simulink model "GolfSwing3D_KineticallyDrivenBlockCountStrip"  (R2024b)
settings: Solver=VariableStepAuto  StartTime=0.0  StopTime=StopTime  MaxStep=0.001  RelTol=1e-3
model workspace: external: MAT-File 3DModelInputs.mat (data not in the file)
undefined symbols (not defined in the file or in its folder): GripStrength, KillswitchFinalValue, KillswitchInitialValue, KillswitchStepTime, LeftLowerArmLength, PlaneTilt, RightLowerArmLength, UpperTorsoLength, X, Y, Z
libraries: nesl_utility x361, sm_lib x136, matrix_library x11, fl_lib x2, simulink x1
(part 12 of 13)

== matlab function GolfSwing3D_KineticallyDrivenBlockCountStrip/RE Input Function/Right Elbow Input Torque ==
  data: Time input; Killswitch input; JointTorqueRE output; REPositionInput output; REInputB parameter; REPositionSetpoint parameter; GlobalGain parameter; REDampening parameter; ModelingMode parameter; GlobalPCGain parameter; GlobalVCGain parameter; DampeningGlobalGain parameter; TargetImpactTime parameter; KinematicMode parameter; REAo parameter; REStartPosition parameter; REStartVelocity parameter; REVCGain parameter; TargetREVelocity parameter; TargetREPosition parameter; REPositionGain parameter; REInputC parameter; RETimeGain parameter; REVelocityInput output; REAccelerationInput output; REConstant parameter; REPosition input; REVelocity input; ZVCFRETorque parameter; REPCGain parameter; REInputA parameter; REAf parameter; REInputD parameter; REInputE parameter; REInputF parameter; REInputG parameter
function [JointTorqueRE,REPositionInput,REVelocityInput,...
    REAccelerationInput]  = fcn(Time,Killswitch,...
    REInputB,REPositionSetpoint,GlobalGain,...
    REDampening, ModelingMode,GlobalPCGain, GlobalVCGain,...
    DampeningGlobalGain,TargetImpactTime,KinematicMode, REAo,REStartPosition,...
    REStartVelocity,REVCGain,...
    TargetREVelocity,TargetREPosition, ...
    REPositionGain,REInputC,...
    RETimeGain, REConstant, REPosition,REVelocity, ZVCFRETorque, REPCGain,...
    REInputA,REAf,REInputD, REInputE, REInputF, REInputG)

%Tau=Time/TargetImpactTime;
t=Time;

% %%%%%%%%%%%%%%%%%%%%%%%%%%%%%%%%%%%%%%%%%%%
% % Kinetic Input Selection and Calculation
% %%%%%%%%%%%%%%%%%%%%%%%%%%%%%%%%%%%%%%%%%%%

if ModelingMode==0
    % Values are all set to zero.
    JointTorqueRE=0;
elseif ModelingMode==1
    % Control based strategy. Values are based on difference in value
    % between the current state and desired state.
    % RE Joint Rotational Deltas
    DeltaREPosition=REPosition-TargetREPosition;
    DeltaREVelocity=REVelocity-TargetREVelocity;
    % Control Based Strategy
    JointTorqueRE=DeltaREPosition*REPCGain*GlobalPCGain-DeltaREVelocity*REVCGain*GlobalVCGain-DampeningGlobalGain*REDampening*REVelocity;
elseif ModelingMode==2
    % Forward Dynamics Based Strategy. Values are computed based on a
    % polynomial and a combination of dampening and position gained
    % factors.
    JointTorqueRE=Killswitch*GlobalGain*(REConstant+RETimeGain*Time-REPositionGain*(REPosition-REPositionSetpoint)...
    -REDampening*REVelocity);
elseif ModelingMode==3
    JointTorqueRE=HexPolyInputFunction(REInputA,REInputB,REInputC,REInputD,REInputE,REInputF,REInputG,Time)*Killswitch;
else
    %ZVCF Based Joint Torques. Values are pulled from model workspace and
    %held constant.
    JointTorqueRE=ZVCFRETorque;
end

% %%%%%%%%%%%%%%%%%%%%%%%%%%%%%%%%%%%%%%%%%%%
% % Kinematic Input Selection and Calculation
% %%%%%%%%%%%%%%%%%%%%%%%%%%%%%%%%%%%%%%%%%%%

% Manual Set Option
% KinematicMode=3;

if KinematicMode==0
    % All kinematic values set to zero.
    REPositionInput=0;
    REVelocityInput=0;
    REAccelerationInput=0;
elseif KinematicMode==1
    % 1st Order Acceleration, 2nd Order Velocity, 3rd Order Position Solution
    PTX=TargetREPosition;       
    VTX=TargetREVelocity;
    % Define Starting Position and Velocity
    PIX=REStartPosition;
    VIX=REStartVelocity;
    AX=3*((VTX+VIX)*TargetImpactTime-2*(PTX-PIX))/TargetImpactTime^3;         % Constant in position equation
    BX=-2*((VTX+2*VIX)*TargetImpactTime-3*(PTX-PIX))/TargetImpactTime^2;         % Constant in position equation
    CX=VIX;         % Starting Velocity at Time Zero
    DX=PIX;         % Starting Position at Time Zero
    % Equation for position as a function of time
    REPositionInput=AX*Time^3/3+BX*Time^2/2+CX*Time+DX;
    REVelocityInput=AX*Time^2+BX*Time+CX;
    REAccelerationInput=2*AX*Time+BX;
elseif KinematicMode==2
    % 2nd Order Acceleration, 3rd Order Velocity, 4th Order Position Solution
    Tt=TargetImpactTime;
    t=Time;
    PoX=REStartPosition;
    VoX=REStartVelocity;
    PfX=TargetREPosition;
    VfX=TargetREVelocity;
    AoX=REAo;
    REPositionInput=PoX + VoX*t + (AoX*t^2)/2 - (t^3*(4*PoX - 4*PfX + Tt*VfX + 3*Tt*VoX + AoX*Tt^2))/Tt^3 + (t^4*(6*PoX - 6*PfX + 2*Tt*VfX + 4*Tt*VoX + AoX*Tt^2))/(2*Tt^4);
    REVelocityInput=VoX + AoX*t - (3*t^2*(4*PoX - 4*PfX + Tt*VfX + 3*Tt*VoX + AoX*Tt^2))/Tt^3 + (2*t^3*(6*PoX - 6*PfX + 2*Tt*VfX + 4*Tt*VoX + AoX*Tt^2))/Tt^4;
    REAccelerationInput=AoX + (6*t^2*(6*PoX - 6*PfX + 2*Tt*VfX + 4*Tt*VoX + AoX*Tt^2))/Tt^4 - (6*t*(4*PoX - 4*PfX + Tt*VfX + 3*Tt*VoX + AoX*Tt^2))/Tt^3;
else
    % 3rd Order Acceleration, 4th Order Velocity, 5th Order Position Solution
    Tt=TargetImpactTime;
    t=Time;
    PoX=REStartPosition;
    VoX=REStartVelocity;
    PfX=TargetREPosition;
    VfX=TargetREVelocity;
    AoX=REAo;
    AfX=REAf;
    REPositionInput=PoX+VoX*t+(AoX*t^2)/2-(t^5*(12*PoX-12*PfX+6*Tt*VfX+6*Tt*VoX-AfX*Tt^2+AoX*Tt^2))/(2*Tt^5)-(t^3*(20*PoX-20*PfX+8*Tt*VfX+12*Tt*VoX-AfX*Tt^2+3*AoX*Tt^2))/(2*Tt^3)+(t^4*(30*PoX-30*PfX+14*Tt*VfX+16*Tt*VoX-2*AfX*Tt^2+3*AoX*Tt^2))/(2*Tt^4);
    REVelocityInput=VoX+AoX*t-(5*t^4*(12*PoX-12*PfX+6*Tt*VfX+6*Tt*VoX-AfX*Tt^2+AoX*Tt^2))/(2*Tt^5)-(3*t^2*(20*PoX-20*PfX+8*Tt*VfX+12*Tt*VoX-AfX*Tt^2+3*AoX*Tt^2))/(2*Tt^3)+(2*t^3*(30*PoX-30*PfX+14*Tt*VfX+16*Tt*VoX-2*AfX*Tt^2+3*AoX*Tt^2))/Tt^4;
    REAccelerationInput=AoX-(3*t*(20*PoX-20*PfX+8*Tt*VfX+12*Tt*VoX-AfX*Tt^2+3*AoX*Tt^2))/Tt^3-(10*t^3*(12*PoX-12*PfX+6*Tt*VfX+6*Tt*VoX-AfX*Tt^2+AoX*Tt^2))/Tt^5+(6*t^2*(30*PoX-30*PfX+14*Tt*VfX+16*Tt*VoX-2*AfX*Tt^2+3*AoX*Tt^2))/Tt^4;
end

% Calculate Higher Order Derivatives of the Position Outputs
REJerk=gradient(REAccelerationInput,t);
RESnap=gradient(REJerk,t);
RECrackle=gradient(RESnap,t);
REPop=gradient(RECrackle,t);

== matlab function GolfSwing3D_KineticallyDrivenBlockCountStrip/Right Hand/RW Unit Vector ==
  data: RWv input; RWSpeed output; RWvx input; RWvy input; RWvz input; RWuvx output; RWuvy output; RWuvz output
function [RWSpeed,RWuvx,RWuvy,RWuvz]  = fcn(RWv,RWvx,RWvy,RWvz)

RWSpeed=norm(RWv);
RWuvx=RWvx/RWSpeed;
RWuvy=RWvy/RWSpeed;
RWuvz=RWvz/RWSpeed;

== matlab function GolfSwing3D_KineticallyDrivenBlockCountStrip/LF Input Function/LF Input Torque ==
  data: Time input; Killswitch input; JointTorqueLF output; LFPositionInput output; LFInputB parameter; LFPositionSetpoint parameter; GlobalGain parameter; LFDampening parameter; ModelingMode parameter; GlobalPCGain parameter; GlobalVCGain parameter; DampeningGlobalGain parameter; TargetImpactTime parameter; KinematicMode parameter; LFAo parameter; LFStartPosition parameter; LFStartVelocity parameter; LFVCGain parameter; TargetLFVelocity parameter; TargetLFPosition parameter; LFPositionGain parameter; LFInputC parameter; LFTimeGain parameter; LFVelocityInput output; LFAccelerationInput output; LFConstant parameter; LFPosition input; LFVelocity input; ZVCFLFTorque parameter; LFPCGain parameter; LFInputA parameter; LFAf parameter; LFInputD parameter; LFInputE parameter; LFInputF parameter; LFInputG parameter
function [JointTorqueLF,LFPositionInput,LFVelocityInput,...
    LFAccelerationInput]  = fcn(Time,Killswitch,...
    LFInputB,LFPositionSetpoint,GlobalGain,...
    LFDampening, ModelingMode,GlobalPCGain, GlobalVCGain,...
    DampeningGlobalGain,TargetImpactTime,KinematicMode, LFAo,LFStartPosition,...
    LFStartVelocity,LFVCGain,...
    TargetLFVelocity,TargetLFPosition, ...
    LFPositionGain,LFInputC,...
    LFTimeGain, LFConstant, LFPosition,LFVelocity, ZVCFLFTorque, LFPCGain,...
    LFInputA,LFAf, LFInputD, LFInputE, LFInputF, LFInputG)

%Tau=Time/TargetImpactTime;
t=Time;

% %%%%%%%%%%%%%%%%%%%%%%%%%%%%%%%%%%%%%%%%%%%
% % Kinetic Input Selection and Calculation
% %%%%%%%%%%%%%%%%%%%%%%%%%%%%%%%%%%%%%%%%%%%

if ModelingMode==0
    % Values are all set to zero.
    JointTorqueLF=0;
elseif ModelingMode==1
    % Control based strategy. Values are based on difference in value
    % between the current state and desired state.
    % LF Joint Rotational Deltas
    DeltaLFPosition=LFPosition-TargetLFPosition;
    DeltaLFVelocity=LFVelocity-TargetLFVelocity;
    % Control Based Strategy
    JointTorqueLF=DeltaLFPosition*LFPCGain*GlobalPCGain-DeltaLFVelocity*LFVCGain*GlobalVCGain-DampeningGlobalGain*LFDampening*LFVelocity;
elseif ModelingMode==2
    % Forward Dynamics Based Strategy. Values are computed based on a
    % polynomial and a combination of dampening and position gained
    % factors.
    JointTorqueLF=Killswitch*GlobalGain*(LFConstant+LFTimeGain*Time-LFPositionGain*(LFPosition-LFPositionSetpoint)...
    -LFDampening*LFVelocity);
elseif ModelingMode==3
    JointTorqueLF=HexPolyInputFunction(LFInputA,LFInputB,LFInputC,LFInputD,LFInputE,LFInputF,LFInputG,Time)*Killswitch;
else
    %ZVCF Based Joint Torques. Values are pulled from model workspace and
    %held constant.
    JointTorqueLF=ZVCFLFTorque;
end

% %%%%%%%%%%%%%%%%%%%%%%%%%%%%%%%%%%%%%%%%%%%
% % Kinematic Input Selection and Calculation
% %%%%%%%%%%%%%%%%%%%%%%%%%%%%%%%%%%%%%%%%%%%

if KinematicMode==0
    % All kinematic values set to zero.
    LFPositionInput=0;
    LFVelocityInput=0;
    LFAccelerationInput=0;
elseif KinematicMode==1
    % 1st Order Acceleration, 2nd Order Velocity, 3rd Order Position Solution
    PTX=TargetLFPosition;       
    VTX=TargetLFVelocity;
    % Define Starting Position and Velocity
    PIX=LFStartPosition;
    VIX=LFStartVelocity;
    AX=3*((VTX+VIX)*TargetImpactTime-2*(PTX-PIX))/TargetImpactTime^3;         % Constant in position equation
    BX=-2*((VTX+2*VIX)*TargetImpactTime-3*(PTX-PIX))/TargetImpactTime^2;         % Constant in position equation
    CX=VIX;         % Starting Velocity at Time Zero
    DX=PIX;         % Starting Position at Time Zero
    % Equation for position as a function of time
    LFPositionInput=AX*Time^3/3+BX*Time^2/2+CX*Time+DX;
    LFVelocityInput=AX*Time^2+BX*Time+CX;
    LFAccelerationInput=2*AX*Time+BX;
elseif KinematicMode==2
    % 2nd Order Acceleration, 3rd Order Velocity, 4th Order Position Solution
    Tt=TargetImpactTime;
    t=Time;
    PoX=LFStartPosition;
    VoX=LFStartVelocity;
    PfX=TargetLFPosition;
    VfX=TargetLFVelocity;
    AoX=LFAo;
    LFPositionInput=PoX + VoX*t + (AoX*t^2)/2 - (t^3*(4*PoX - 4*PfX + Tt*VfX + 3*Tt*VoX + AoX*Tt^2))/Tt^3 + (t^4*(6*PoX - 6*PfX + 2*Tt*VfX + 4*Tt*VoX + AoX*Tt^2))/(2*Tt^4);
    LFVelocityInput=VoX + AoX*t - (3*t^2*(4*PoX - 4*PfX + Tt*VfX + 3*Tt*VoX + AoX*Tt^2))/Tt^3 + (2*t^3*(6*PoX - 6*PfX + 2*Tt*VfX + 4*Tt*VoX + AoX*Tt^2))/Tt^4;
    LFAccelerationInput=AoX + (6*t^2*(6*PoX - 6*PfX + 2*Tt*VfX + 4*Tt*VoX + AoX*Tt^2))/Tt^4 - (6*t*(4*PoX - 4*PfX + Tt*VfX + 3*Tt*VoX + AoX*Tt^2))/Tt^3;
else
    % 3rd Order Acceleration, 4th Order Velocity, 5th Order Position Solution
    Tt=TargetImpactTime;
    t=Time;
    PoX=LFStartPosition;
    VoX=LFStartVelocity;
    PfX=TargetLFPosition;
    VfX=TargetLFVelocity;
    AoX=LFAo;
    AfX=LFAf;
    LFPositionInput=PoX+VoX*t+(AoX*t^2)/2-(t^5*(12*PoX-12*PfX+6*Tt*VfX+6*Tt*VoX-AfX*Tt^2+AoX*Tt^2))/(2*Tt^5)-(t^3*(20*PoX-20*PfX+8*Tt*VfX+12*Tt*VoX-AfX*Tt^2+3*AoX*Tt^2))/(2*Tt^3)+(t^4*(30*PoX-30*PfX+14*Tt*VfX+16*Tt*VoX-2*AfX*Tt^2+3*AoX*Tt^2))/(2*Tt^4);
    LFVelocityInput=VoX+AoX*t-(5*t^4*(12*PoX-12*PfX+6*Tt*VfX+6*Tt*VoX-AfX*Tt^2+AoX*Tt^2))/(2*Tt^5)-(3*t^2*(20*PoX-20*PfX+8*Tt*VfX+12*Tt*VoX-AfX*Tt^2+3*AoX*Tt^2))/(2*Tt^3)+(2*t^3*(30*PoX-30*PfX+14*Tt*VfX+16*Tt*VoX-2*AfX*Tt^2+3*AoX*Tt^2))/Tt^4;
    LFAccelerationInput=AoX-(3*t*(20*PoX-20*PfX+8*Tt*VfX+12*Tt*VoX-AfX*Tt^2+3*AoX*Tt^2))/Tt^3-(10*t^3*(12*PoX-12*PfX+6*Tt*VfX+6*Tt*VoX-AfX*Tt^2+AoX*Tt^2))/Tt^5+(6*t^2*(30*PoX-30*PfX+14*Tt*VfX+16*Tt*VoX-2*AfX*Tt^2+3*AoX*Tt^2))/Tt^4;
end

% Calculate Higher Order Derivatives of the Position Outputs
LFJerk=gradient(LFAccelerationInput,t);
LFSnap=gradient(LFJerk,t);
LFCrackle=gradient(LFSnap,t);
LFPop=gradient(LFCrackle,t);

== matlab function GolfSwing3D_KineticallyDrivenBlockCountStrip/Translation Input Function/GlobalBaseTranslationalForce ==
  data: Time input; Killswitch input; TranslationInputXA parameter; TranslationInputYA parameter; TranslationInputZA parameter; TranslationInputXB parameter; TranslationInputYB parameter; TranslationInputZB parameter; TranslationPositionSetpointX parameter; TranslationPositionSetpointY parameter; GlobalGain parameter; TranslationForceX output; TranslationForceY output; TranslationForceZ output; TranslationDampeningX parameter; TranslationDampeningY parameter; TranslationDampeningZ parameter; TranslationConstantX parameter; TranslationConstantY parameter; TranslationConstantZ parameter; TranslationTimeGainX parameter; TranslationPositionGainY parameter; TranslationPositionGainZ parameter; TranslationPositionSetpointZ parameter; TargetTranslationPositionX parameter; TargetTranslationPositionY parameter; TargetTranslationPositionZ parameter; TargetTranslationVelocityX parameter; TargetTranslationVelocityY parameter; TargetTranslationVelocityZ parameter; TranslationPCGainX parameter; TranslationPCGainY parameter; TranslationPCGainZ parameter; TranslationVCGainX parameter; TranslationVCGainY parameter; TranslationVCGainZ parameter; ModelingMode parameter; ZVCFTranslationForceX parameter; ZVCFTranslationForceY parameter; ZVCFTranslationForceZ parameter; GlobalPCGain parameter; GlobalVCGain parameter; DampeningGlobalGain parameter; TargetImpactTime parameter; TranslationStartPositionX parameter; TranslationPositionInputX output; TranslationPositionInputY output; TranslationPositionInputZ output; TranslationVelocityInputX output; TranslationVelocityInputY output; TranslationVelocityInputZ output; TranslationAccelerationInputX output; TranslationAccelerationInputY output; TranslationAccelerationInputZ output; TranslationStartPositionY parameter; TranslationStartPositionZ parameter; TranslationStartVelocityX parameter; TranslationStartVelocityY parameter; TranslationStartVelocityZ parameter; TranslationPositionX input; TranslationPositionY input; TranslationPositionZ input; TranslationInputYC parameter; TranslationInputZC parameter; TranslationInputXC parameter; TranslationAoX parameter; TranslationAoY parameter; TranslationAoZ parameter; TranslationPositionGainX parameter; TranslationTimeGainY parameter; TranslationTimeGainZ parameter; TranslationVelocityX input; TranslationVelocityY input; TranslationVelocityZ input; KinematicMode parameter; TranslationAfX parameter; TranslationAfY parameter; TranslationAfZ parameter; TranslationInputXD parameter; TranslationInputXE parameter; TranslationInputXF parameter; TranslationInputXG parameter; TranslationInputYD parameter; TranslationInputYE parameter; TranslationInputYF parameter; TranslationInputYG parameter; TranslationInputZD parameter; TranslationInputZE parameter; TranslationInputZF parameter; TranslationInputZG parameter
function [TranslationForceX,TranslationForceY,TranslationForceZ,TranslationPositionInputX,TranslationPositionInputY,TranslationPositionInputZ,TranslationVelocityInputX,...
    TranslationVelocityInputY, TranslationVelocityInputZ,TranslationAccelerationInputX,TranslationAccelerationInputY,TranslationAccelerationInputZ] = fcn(Time,Killswitch, TranslationInputXA,TranslationInputYA,TranslationInputZA,TranslationInputXB,TranslationInputYB,TranslationInputZB, TranslationPositionSetpointX,TranslationPositionSetpointY,GlobalGain,...
    TranslationDampeningX, TranslationDampeningY, TranslationDampeningZ, TranslationConstantX, TranslationConstantY, TranslationConstantZ, TranslationTimeGainX, TranslationPositionGainY, TranslationPositionGainZ, TranslationPositionSetpointZ,...
    TargetTranslationPositionX, TargetTranslationPositionY, TargetTranslationPositionZ, TargetTranslationVelocityX, TargetTranslationVelocityY, TargetTranslationVelocityZ,TranslationPCGainX, TranslationPCGainY, TranslationPCGainZ, TranslationVCGainX,...
    TranslationVCGainY, TranslationVCGainZ,ModelingMode,ZVCFTranslationForceX, ZVCFTranslationForceY, ZVCFTranslationForceZ,GlobalPCGain, GlobalVCGain,DampeningGlobalGain,TargetImpactTime,TranslationStartPositionX,...
    TranslationStartPositionY, TranslationStartPositionZ, TranslationStartVelocityX, TranslationStartVelocityY, TranslationStartVelocityZ,TranslationPositionX, TranslationPositionY, TranslationPositionZ, TranslationInputYC, TranslationInputZC,...
TranslationInputXC, TranslationAoX, TranslationAoY, TranslationAoZ, TranslationPositionGainX, TranslationTimeGainY, TranslationTimeGainZ, TranslationVelocityX, TranslationVelocityY,...
TranslationVelocityZ,KinematicMode, TranslationAfX, TranslationAfY, TranslationAfZ,TranslationInputXD, TranslationInputXE, TranslationInputXF, TranslationInputXG, TranslationInputYD,...
TranslationInputYE, TranslationInputYF, TranslationInputYG, TranslationInputZD, TranslationInputZE, TranslationInputZF, TranslationInputZG)

%Tau=Time/TargetImpactTime;
t=Time;

% %%%%%%%%%%%%%%%%%%%%%%%%%%%%%%%%%%%%%%%%%%%
% % Kinetic Input Selection and Calculation
% %%%%%%%%%%%%%%%%%%%%%%%%%%%%%%%%%%%%%%%%%%%

if ModelingMode==0
    % Values are all set to zero.
    TranslationForceX=0;
    TranslationForceY=0;
    TranslationForceZ=0;
elseif ModelingMode==1
    % Control based strategy. Values are based on difference in value
    % between the current state and desired state.
    % Translation Joint Rotational Deltas
    DeltaTranslationPositionX=TranslationPositionX-TargetTranslationPositionX;
    DeltaTranslationPositionY=TranslationPositionY-TargetTranslationPositionY;
    DeltaTranslationPositionZ=TranslationPositionZ-TargetTranslationPositionZ;
    DeltaTranslationVelocityX=TranslationVelocityX-TargetTranslationVelocityX;
    DeltaTranslationVelocityY=TranslationVelocityY-TargetTranslationVelocityY;
    DeltaTranslationVelocityZ=TranslationVelocityZ-TargetTranslationVelocityZ;
    % Control Based Strategy
    TranslationForceX=DeltaTranslationPositionX*TranslationPCGainX*GlobalPCGain-DeltaTranslationVelocityX*TranslationVCGainX*GlobalVCGain-DampeningGlobalGain*TranslationDampeningX*TranslationVelocityX;
    TranslationForceY=DeltaTranslationPositionY*TranslationPCGainY*GlobalPCGain-DeltaTranslationVelocityY*TranslationVCGainY*GlobalVCGain-DampeningGlobalGain*TranslationDampeningY*TranslationVelocityY;
    TranslationForceZ=DeltaTranslationPositionZ*TranslationPCGainZ*GlobalPCGain-DeltaTranslationVelocityZ*TranslationVCGainZ*GlobalVCGain-DampeningGlobalGain*TranslationDampeningZ*TranslationVelocityZ;
elseif ModelingMode==2
    % Forward Dynamics Based Strategy. Values are computed based on a
    % polynomial and a combination of dampening and position gained
    % factors.
    TranslationForceX=Killswitch*GlobalGain*(TranslationConstantX+TranslationTimeGainX*Time-TranslationPositionGainX*(TranslationPositionX-TranslationPositionSetpointX)...
    -TranslationDampeningX*TranslationVelocityX);
    TranslationForceY=Killswitch*GlobalGain*(TranslationConstantY+TranslationTimeGainY*Time-TranslationPositionGainY*(TranslationPositionY-TranslationPositionSetpointY)...
    -TranslationDampeningY*TranslationVelocityY);
    TranslationForceZ=Killswitch*GlobalGain*(TranslationConstantZ+TranslationTimeGainZ*Time-TranslationPositionGainZ*(TranslationPositionZ-TranslationPositionSetpointZ)...
    -TranslationDampeningZ*TranslationVelocityZ);
elseif ModelingMode==3
    TranslationForceX=HexPolyInputFunction(TranslationInputXA,TranslationInputXB,TranslationInputXC,TranslationInputXD,TranslationInputXE,TranslationInputXF,TranslationInputXG,Time)*Killswitch;
    TranslationForceY=HexPolyInputFunction(TranslationInputYA,TranslationInputYB,TranslationInputYC,TranslationInputYD,TranslationInputYE,TranslationInputYF,TranslationInputYG,Time)*Killswitch;
    TranslationForceZ=HexPolyInputFunction(TranslationInputZA,TranslationInputZB,TranslationInputZC,TranslationInputZD,TranslationInputZE,TranslationInputZF,TranslationInputZG,Time)*Killswitch;
else
    %ZVCF Based Joint Forces. Values are pulled from model workspace and
    %held constant.
    TranslationForceX=ZVCFTranslationForceX;
    TranslationForceY=ZVCFTranslationForceY;
    TranslationForceZ=ZVCFTranslationForceZ;
end

% %%%%%%%%%%%%%%%%%%%%%%%%%%%%%%%%%%%%%%%%%%%
% % Kinematic Input Selection and Calculation
% %%%%%%%%%%%%%%%%%%%%%%%%%%%%%%%%%%%%%%%%%%%

if KinematicMode==0
    % All kinematic values set to zero.
    TranslationPositionInputX=0;
    TranslationPositionInputY=0;
    TranslationPositionInputZ=0;
    TranslationVelocityInputX=0;
    TranslationVelocityInputY=0;
    TranslationVelocityInputZ=0;
    TranslationAccelerationInputX=0;
    TranslationAccelerationInputY=0;
    TranslationAccelerationInputZ=0;
elseif KinematicMode==1
    % 1st Order Acceleration, 2nd Order Velocity, 3rd Order Position Solution
    PTX=TargetTranslationPositionX;       
    VTX=TargetTranslationVelocityX;
    PTY=TargetTranslationPositionY;
    VTY=TargetTranslationVelocityY;
    PTZ=TargetTranslationPositionZ;
    VTZ=TargetTranslationVelocityZ;
    % Define Starting Position and Velocity
    PIX=TranslationStartPositionX;
    VIX=TranslationStartVelocityX;
    PIY=TranslationStartPositionY;
    VIY=TranslationStartVelocityY;
    PIZ=TranslationStartPositionZ;
    VIZ=TranslationStartVelocityZ;
    AX=3*((VTX+VIX)*TargetImpactTime-2*(PTX-PIX))/TargetImpactTime^3;         % Constant in position equation
    BX=-2*((VTX+2*VIX)*TargetImpactTime-3*(PTX-PIX))/TargetImpactTime^2;         % Constant in position equation
    CX=VIX;         % Starting Velocity at Time Zero
    DX=PIX;         % Starting Position at Time Zero
    AY=3*((VTY+VIY)*TargetImpactTime-2*(PTY-PIY))/TargetImpactTime^3;         % Constant in position equation
    BY=-2*((VTY+2*VIY)*TargetImpactTime-3*(PTY-PIY))/TargetImpactTime^2;         % Constant in position equation
    CY=VIY;         % Starting Velocity at Time Zero
    DY=PIY;         % Starting Position at Time Zero
    AZ=3*((VTZ+VIZ)*TargetImpactTime-2*(PTZ-PIZ))/TargetImpactTime^3;         % Constant in position equation
    BZ=-2*((VTZ+2*VIZ)*TargetImpactTime-3*(PTZ-PIZ))/TargetImpactTime^2;         % Constant in position equation
    CZ=VIZ;         % Starting Velocity at Time Zero
    DZ=PIZ;         % Starting Position at Time Zero
    % Equation for position as a function of time
    TranslationPositionInputX=AX*Time^3/3+BX*Time^2/2+CX*Time+DX;
    TranslationPositionInputY=AY*Time^3/3+BY*Time^2/2+CY*Time+DY;
    TranslationPositionInputZ=AZ*Time^3/3+BZ*Time^2/2+CZ*Time+DZ;
    TranslationVelocityInputX=AX*Time^2+BX*Time+CX;
    TranslationVelocityInputY=AY*Time^2+BY*Time+CY;
    TranslationVelocityInputZ=AZ*Time^2+BZ*Time+CZ;
    TranslationAccelerationInputX=2*AX*Time+BX;
    TranslationAccelerationInputY=2*AY*Time+BY;
    TranslationAccelerationInputZ=2*AZ*Time+BZ;
elseif KinematicMode==2
    % 2nd Order Acceleration, 3rd Order Velocity, 4th Order Position Solution
    Tt=TargetImpactTime;
    t=Time;
    PoX=TranslationStartPositionX;
    PoY=TranslationStartPositionY;
    PoZ=TranslationStartPositionZ;
    VoX=TranslationStartVelocityX;
    VoY=TranslationStartVelocityY;
    VoZ=TranslationStartVelocityZ;
    PfX=TargetTranslationPositionX;
    PfY=TargetTranslationPositionY;
    PfZ=TargetTranslationPositionZ;
    VfX=TargetTranslationVelocityX;
    VfY=TargetTranslationVelocityY;
    VfZ=TargetTranslationVelocityZ;
    AoX=TranslationAoX;
    AoY=TranslationAoY;
    AoZ=TranslationAoZ;
    TranslationPositionInputX=PoX + VoX*t + (AoX*t^2)/2 - (t^3*(4*PoX - 4*PfX + Tt*VfX + 3*Tt*VoX + AoX*Tt^2))/Tt^3 + (t^4*(6*PoX - 6*PfX + 2*Tt*VfX + 4*Tt*VoX + AoX*Tt^2))/(2*Tt^4);
    TranslationPositionInputY=PoY + VoY*t + (AoY*t^2)/2 - (t^3*(4*PoY - 4*PfY + Tt*VfY + 3*Tt*VoY + AoY*Tt^2))/Tt^3 + (t^4*(6*PoY - 6*PfY + 2*Tt*VfY + 4*Tt*VoY + AoY*Tt^2))/(2*Tt^4);
    TranslationPositionInputZ=PoZ + VoZ*t + (AoZ*t^2)/2 - (t^3*(4*PoZ - 4*PfZ + Tt*VfZ + 3*Tt*VoZ + AoZ*Tt^2))/Tt^3 + (t^4*(6*PoZ - 6*PfZ + 2*Tt*VfZ + 4*Tt*VoZ + AoZ*Tt^2))/(2*Tt^4);
    TranslationVelocityInputX=VoX + AoX*t - (3*t^2*(4*PoX - 4*PfX + Tt*VfX + 3*Tt*VoX + AoX*Tt^2))/Tt^3 + (2*t^3*(6*PoX - 6*PfX + 2*Tt*VfX + 4*Tt*VoX + AoX*Tt^2))/Tt^4;
    TranslationVelocityInputY=VoY + AoY*t - (3*t^2*(4*PoY - 4*PfY + Tt*VfY + 3*Tt*VoY + AoY*Tt^2))/Tt^3 + (2*t^3*(6*PoY - 6*PfY + 2*Tt*VfY + 4*Tt*VoY + AoY*Tt^2))/Tt^4;
    TranslationVelocityInputZ=VoZ + AoZ*t - (3*t^2*(4*PoZ - 4*PfZ + Tt*VfZ + 3*Tt*VoZ + AoZ*Tt^2))/Tt^3 + (2*t^3*(6*PoZ - 6*PfZ + 2*Tt*VfZ + 4*Tt*VoZ + AoZ*Tt^2))/Tt^4;
    TranslationAccelerationInputX=AoX + (6*t^2*(6*PoX - 6*PfX + 2*Tt*VfX + 4*Tt*VoX + AoX*Tt^2))/Tt^4 - (6*t*(4*PoX - 4*PfX + Tt*VfX + 3*Tt*VoX + AoX*Tt^2))/Tt^3;
    TranslationAccelerationInputY=AoY + (6*t^2*(6*PoY - 6*PfY + 2*Tt*VfY + 4*Tt*VoY + AoY*Tt^2))/Tt^4 - (6*t*(4*PoY - 4*PfY + Tt*VfY + 3*Tt*VoY + AoY*Tt^2))/Tt^3;
    TranslationAccelerationInputZ=AoZ + (6*t^2*(6*PoZ - 6*PfZ + 2*Tt*VfZ + 4*Tt*VoZ + AoZ*Tt^2))/Tt^4 - (6*t*(4*PoZ - 4*PfZ + Tt*VfZ + 3*Tt*VoZ + AoZ*Tt^2))/Tt^3;
else
    % 3rd Order Acceleration, 4th Order Velocity, 5th Order Position Solution
    Tt=TargetImpactTime;
    t=Time;
    PoX=TranslationStartPositionX;
    PoY=TranslationStartPositionY;
    PoZ=TranslationStartPositionZ;
    VoX=TranslationStartVelocityX;
    VoY=TranslationStartVelocityY;
    VoZ=TranslationStartVelocityZ;
    PfX=TargetTranslationPositionX;
    PfY=TargetTranslationPositionY;
    PfZ=TargetTranslationPositionZ;
    VfX=TargetTranslationVelocityX;
    VfY=TargetTranslationVelocityY;
    VfZ=TargetTranslationVelocityZ;
    AoX=TranslationAoX;
    AoY=TranslationAoY;
    AoZ=TranslationAoZ;
    AfX=TranslationAfX;
    AfY=TranslationAfY;
    AfZ=TranslationAfZ;
    TranslationPositionInputX=PoX+VoX*t+(AoX*t^2)/2-(t^5*(12*PoX-12*PfX+6*Tt*VfX+6*Tt*VoX-AfX*Tt^2+AoX*Tt^2))/(2*Tt^5)-(t^3*(20*PoX-20*PfX+8*Tt*VfX+12*Tt*VoX-AfX*Tt^2+3*AoX*Tt^2))/(2*Tt^3)+(t^4*(30*PoX-30*PfX+14*Tt*VfX+16*Tt*VoX-2*AfX*Tt^2+3*AoX*Tt^2))/(2*Tt^4);
    TranslationPositionInputY=PoY+VoY*t+(AoY*t^2)/2-(t^5*(12*PoY-12*PfY+6*Tt*VfY+6*Tt*VoY-AfY*Tt^2+AoY*Tt^2))/(2*Tt^5)-(t^3*(20*PoY-20*PfY+8*Tt*VfY+12*Tt*VoY-AfY*Tt^2+3*AoY*Tt^2))/(2*Tt^3)+(t^4*(30*PoY-30*PfY+14*Tt*VfY+16*Tt*VoY-2*AfY*Tt^2+3*AoY*Tt^2))/(2*Tt^4);  
    TranslationPositionInputZ=PoZ+VoZ*t+(AoZ*t^2)/2-(t^5*(12*PoZ-12*PfZ+6*Tt*VfZ+6*Tt*VoZ-AfZ*Tt^2+AoZ*Tt^2))/(2*Tt^5)-(t^3*(20*PoZ-20*PfZ+8*Tt*VfZ+12*Tt*VoZ-AfZ*Tt^2+3*AoZ*Tt^2))/(2*Tt^3)+(t^4*(30*PoZ-30*PfZ+14*Tt*VfZ+16*Tt*VoZ-2*AfZ*Tt^2+3*AoZ*Tt^2))/(2*Tt^4);
    TranslationVelocityInputX=VoX+AoX*t-(5*t^4*(12*PoX-12*PfX+6*Tt*VfX+6*Tt*VoX-AfX*Tt^2+AoX*Tt^2))/(2*Tt^5)-(3*t^2*(20*PoX-20*PfX+8*Tt*VfX+12*Tt*VoX-AfX*Tt^2+3*AoX*Tt^2))/(2*Tt^3)+(2*t^3*(30*PoX-30*PfX+14*Tt*VfX+16*Tt*VoX-2*AfX*Tt^2+3*AoX*Tt^2))/Tt^4;
    TranslationVelocityInputY=VoY+AoY*t-(5*t^4*(12*PoY-12*PfY+6*Tt*VfY+6*Tt*VoY-AfY*Tt^2+AoY*Tt^2))/(2*Tt^5)-(3*t^2*(20*PoY-20*PfY+8*Tt*VfY+12*Tt*VoY-AfY*Tt^2+3*AoY*Tt^2))/(2*Tt^3)+(2*t^3*(30*PoY-30*PfY+14*Tt*VfY+16*Tt*VoY-2*AfY*Tt^2+3*AoY*Tt^2))/Tt^4;
    TranslationVelocityInputZ=VoZ+AoZ*t-(5*t^4*(12*PoZ-12*PfZ+6*Tt*VfZ+6*Tt*VoZ-AfZ*Tt^2+AoZ*Tt^2))/(2*Tt^5)-(3*t^2*(20*PoZ-20*PfZ+8*Tt*VfZ+12*Tt*VoZ-AfZ*Tt^2+3*AoZ*Tt^2))/(2*Tt^3)+(2*t^3*(30*PoZ-30*PfZ+14*Tt*VfZ+16*Tt*VoZ-2*AfZ*Tt^2+3*AoZ*Tt^2))/Tt^4;
    TranslationAccelerationInputX=AoX-(3*t*(20*PoX-20*PfX+8*Tt*VfX+12*Tt*VoX-AfX*Tt^2+3*AoX*Tt^2))/Tt^3-(10*t^3*(12*PoX-12*PfX+6*Tt*VfX+6*Tt*VoX-AfX*Tt^2+AoX*Tt^2))/Tt^5+(6*t^2*(30*PoX-30*PfX+14*Tt*VfX+16*Tt*VoX-2*AfX*Tt^2+3*AoX*Tt^2))/Tt^4;
    TranslationAccelerationInputY=AoY-(3*t*(20*PoY-20*PfY+8*Tt*VfY+12*Tt*VoY-AfY*Tt^2+3*AoY*Tt^2))/Tt^3-(10*t^3*(12*PoY-12*PfY+6*Tt*VfY+6*Tt*VoY-AfY*Tt^2+AoY*Tt^2))/Tt^5+(6*t^2*(30*PoY-30*PfY+14*Tt*VfY+16*Tt*VoY-2*AfY*Tt^2+3*AoY*Tt^2))/Tt^4;
    TranslationAccelerationInputZ=AoZ-(3*t*(20*PoZ-20*PfZ+8*Tt*VfZ+12*Tt*VoZ-AfZ*Tt^2+3*AoZ*Tt^2))/Tt^3-(10*t^3*(12*PoZ-12*PfZ+6*Tt*VfZ+6*Tt*VoZ-AfZ*Tt^2+AoZ*Tt^2))/Tt^5+(6*t^2*(30*PoZ-30*PfZ+14*Tt*VfZ+16*Tt*VoZ-2*AfZ*Tt^2+3*AoZ*Tt^2))/Tt^4;
end


% Calculate Higher Order Derivatives of the Position Outputs
TranslationJerkX=gradient(TranslationAccelerationInputX,t);
TranslationJerkY=gradient(TranslationAccelerationInputY,t);
TranslationJerkZ=gradient(TranslationAccelerationInputZ,t);
TranslationSnapX=gradient(TranslationJerkX,t);
TranslationSnapY=gradient(TranslationJerkY,t);
TranslationSnapZ=gradient(TranslationJerkZ,t);
TranslationCrackleX=gradient(TranslationSnapX,t);
TranslationCrackleY=gradient(TranslationSnapY,t);
TranslationCrackleZ=gradient(TranslationSnapZ,t);
TranslationPopX=gradient(TranslationCrackleX,t);
TranslationPopY=gradient(TranslationCrackleY,t);
TranslationPopZ=gradient(TranslationCrackleZ,t);

== matlab function GolfSwing3D_KineticallyDrivenBlockCountStrip/RF Input Function/RF Input Torque ==
  data: Time input; Killswitch input; JointTorqueRF output; RFPositionInput output; RFInputB parameter; RFPositionSetpoint parameter; GlobalGain parameter; RFDampening parameter; ModelingMode parameter; GlobalPCGain parameter; GlobalVCGain parameter; DampeningGlobalGain parameter; TargetImpactTime parameter; KinematicMode parameter; RFAo parameter; RFStartPosition parameter; RFStartVelocity parameter; RFVCGain parameter; TargetRFVelocity parameter; TargetRFPosition parameter; RFPositionGain parameter; RFInputC parameter; RFTimeGain parameter; RFVelocityInput output; RFAccelerationInput output; RFConstant parameter; RFPosition input; RFVelocity input; ZVCFRFTorque parameter; RFPCGain parameter; RFInputA parameter; RFAf parameter; RFInputD parameter; RFInputE parameter; RFInputF parameter; RFInputG parameter
function [JointTorqueRF,RFPositionInput,RFVelocityInput,...
    RFAccelerationInput]  = fcn(Time,Killswitch,...
    RFInputB,RFPositionSetpoint,GlobalGain,...
    RFDampening, ModelingMode,GlobalPCGain, GlobalVCGain,...
    DampeningGlobalGain,TargetImpactTime,KinematicMode, RFAo,RFStartPosition,...
    RFStartVelocity,RFVCGain,...
    TargetRFVelocity,TargetRFPosition, ...
    RFPositionGain,RFInputC,...
    RFTimeGain, RFConstant, RFPosition,RFVelocity, ZVCFRFTorque, RFPCGain,...
    RFInputA,RFAf, RFInputD, RFInputE, RFInputF, RFInputG)

%Tau=Time/TargetImpactTime;
t=Time;

% %%%%%%%%%%%%%%%%%%%%%%%%%%%%%%%%%%%%%%%%%%%
% % Kinetic Input Selection and Calculation
% %%%%%%%%%%%%%%%%%%%%%%%%%%%%%%%%%%%%%%%%%%%

if ModelingMode==0
    % Values are all set to zero.
    JointTorqueRF=0;
elseif ModelingMode==1
    % Control based strategy. Values are based on difference in value
    % between the current state and desired state.
    % RF Joint Rotational Deltas
    DeltaRFPosition=RFPosition-TargetRFPosition;
    DeltaRFVelocity=RFVelocity-TargetRFVelocity;
    % Control Based Strategy
    JointTorqueRF=DeltaRFPosition*RFPCGain*GlobalPCGain-DeltaRFVelocity*RFVCGain*GlobalVCGain-DampeningGlobalGain*RFDampening*RFVelocity;
elseif ModelingMode==2
    % Forward Dynamics Based Strategy. Values are computed based on a
    % polynomial and a combination of dampening and position gained
    % factors.
    JointTorqueRF=Killswitch*GlobalGain*(RFConstant+RFTimeGain*Time-RFPositionGain*(RFPosition-RFPositionSetpoint)...
    -RFDampening*RFVelocity);
elseif ModelingMode==3
    JointTorqueRF=HexPolyInputFunction(RFInputA,RFInputB,RFInputC,RFInputD,RFInputE,RFInputF,RFInputG,Time)*Killswitch;
else
    %ZVCF Based Joint Torques. Values are pulled from model workspace and
    %held constant.
    JointTorqueRF=ZVCFRFTorque;
end

% %%%%%%%%%%%%%%%%%%%%%%%%%%%%%%%%%%%%%%%%%%%
% % Kinematic Input Selection and Calculation
% %%%%%%%%%%%%%%%%%%%%%%%%%%%%%%%%%%%%%%%%%%%

if KinematicMode==0
    % All kinematic values set to zero.
    RFPositionInput=0;
    RFVelocityInput=0;
    RFAccelerationInput=0;
elseif KinematicMode==1
    % 1st Order Acceleration, 2nd Order Velocity, 3rd Order Position Solution
    PTX=TargetRFPosition;       
    VTX=TargetRFVelocity;
    % Define Starting Position and Velocity
    PIX=RFStartPosition;
    VIX=RFStartVelocity;
    AX=3*((VTX+VIX)*TargetImpactTime-2*(PTX-PIX))/TargetImpactTime^3;         % Constant in position equation
    BX=-2*((VTX+2*VIX)*TargetImpactTime-3*(PTX-PIX))/TargetImpactTime^2;         % Constant in position equation
    CX=VIX;         % Starting Velocity at Time Zero
    DX=PIX;         % Starting Position at Time Zero
    % Equation for position as a function of time
    RFPositionInput=AX*Time^3/3+BX*Time^2/2+CX*Time+DX;
    RFVelocityInput=AX*Time^2+BX*Time+CX;
    RFAccelerationInput=2*AX*Time+BX;
elseif KinematicMode==2
    % 2nd Order Acceleration, 3rd Order Velocity, 4th Order Position Solution
    Tt=TargetImpactTime;
    t=Time;
    PoX=RFStartPosition;
    VoX=RFStartVelocity;
    PfX=TargetRFPosition;
    VfX=TargetRFVelocity;
    AoX=RFAo;
    RFPositionInput=PoX + VoX*t + (AoX*t^2)/2 - (t^3*(4*PoX - 4*PfX + Tt*VfX + 3*Tt*VoX + AoX*Tt^2))/Tt^3 + (t^4*(6*PoX - 6*PfX + 2*Tt*VfX + 4*Tt*VoX + AoX*Tt^2))/(2*Tt^4);
    RFVelocityInput=VoX + AoX*t - (3*t^2*(4*PoX - 4*PfX + Tt*VfX + 3*Tt*VoX + AoX*Tt^2))/Tt^3 + (2*t^3*(6*PoX - 6*PfX + 2*Tt*VfX + 4*Tt*VoX + AoX*Tt^2))/Tt^4;
    RFAccelerationInput=AoX + (6*t^2*(6*PoX - 6*PfX + 2*Tt*VfX + 4*Tt*VoX + AoX*Tt^2))/Tt^4 - (6*t*(4*PoX - 4*PfX + Tt*VfX + 3*Tt*VoX + AoX*Tt^2))/Tt^3;
else
    % 3rd Order Acceleration, 4th Order Velocity, 5th Order Position Solution
    Tt=TargetImpactTime;
    t=Time;
    PoX=RFStartPosition;
    VoX=RFStartVelocity;
    PfX=TargetRFPosition;
    VfX=TargetRFVelocity;
    AoX=RFAo;
    AfX=RFAf;
    RFPositionInput=PoX+VoX*t+(AoX*t^2)/2-(t^5*(12*PoX-12*PfX+6*Tt*VfX+6*Tt*VoX-AfX*Tt^2+AoX*Tt^2))/(2*Tt^5)-(t^3*(20*PoX-20*PfX+8*Tt*VfX+12*Tt*VoX-AfX*Tt^2+3*AoX*Tt^2))/(2*Tt^3)+(t^4*(30*PoX-30*PfX+14*Tt*VfX+16*Tt*VoX-2*AfX*Tt^2+3*AoX*Tt^2))/(2*Tt^4);
    RFVelocityInput=VoX+AoX*t-(5*t^4*(12*PoX-12*PfX+6*Tt*VfX+6*Tt*VoX-AfX*Tt^2+AoX*Tt^2))/(2*Tt^5)-(3*t^2*(20*PoX-20*PfX+8*Tt*VfX+12*Tt*VoX-AfX*Tt^2+3*AoX*Tt^2))/(2*Tt^3)+(2*t^3*(30*PoX-30*PfX+14*Tt*VfX+16*Tt*VoX-2*AfX*Tt^2+3*AoX*Tt^2))/Tt^4;
    RFAccelerationInput=AoX-(3*t*(20*PoX-20*PfX+8*Tt*VfX+12*Tt*VoX-AfX*Tt^2+3*AoX*Tt^2))/Tt^3-(10*t^3*(12*PoX-12*PfX+6*Tt*VfX+6*Tt*VoX-AfX*Tt^2+AoX*Tt^2))/Tt^5+(6*t^2*(30*PoX-30*PfX+14*Tt*VfX+16*Tt*VoX-2*AfX*Tt^2+3*AoX*Tt^2))/Tt^4;
end

% Calculate Higher Order Derivatives of the Position Outputs
RFJerk=gradient(RFAccelerationInput,t);
RFSnap=gradient(RFJerk,t);
RFCrackle=gradient(RFSnap,t);
RFPop=gradient(RFCrackle,t);

== matlab function GolfSwing3D_KineticallyDrivenBlockCountStrip/Clubhead/CH Unit Vector ==
  data: CHGlobalPosition input; CHGlobalVelocity input; CHSpeed output; CHSpeedMPH output; CHPathUnitVector output; AoA output; Path output; TipPosition input; Face output; CFUnitVector output; CFVectorLength parameter
function [CHSpeed,CHSpeedMPH,CHPathUnitVector,AoA,Path,Face,CFUnitVector]  = fcn(CHGlobalPosition,CHGlobalVelocity,TipPosition,CFVectorLength)

% Output Blocks for Derivatives: ",dFacedt,dclubfaceuvdt"
% Determine components

CHSpeed=norm(CHGlobalVelocity);
CHuvx=CHGlobalVelocity(1)/CHSpeed;
CHuvy=CHGlobalVelocity(2)/CHSpeed;
CHuvz=CHGlobalVelocity(3)/CHSpeed;
CHPathUnitVector=[CHuvx;CHuvy;CHuvz];

CHSpeedMPH=CHSpeed*2.23694;
CFunitvectorx=(TipPosition(1)-CHGlobalPosition(1))/CFVectorLength;
CFunitvectory=(TipPosition(2)-CHGlobalPosition(2))/CFVectorLength;
CFunitvectorz=(TipPosition(3)-CHGlobalPosition(3))/CFVectorLength;
CFUnitVector=[CFunitvectorx;CFunitvectory;CFunitvectorz];
% Angle of projection of club path to the horizon:
AoA=rad2deg(atan(CHvz/sqrt(CHvx^2+CHvy^2)));

% Angle of the projection of the club path on the ground relative to target
% line:
Path=rad2deg(-atan(CHvy/CHvx));

% Angle of the projection of the clubface unit vector on ground relative to
% target line:
Face=rad2deg(-atan(CFunitvectory/CFunitvectorx));

% dfacedt is magnitude of derivative of the clubface horizontal vector:
% dfacedt=norm(diff(Face));

% dclubfaceuvdt is magnitude of derivative of the clubface unit vector:
% dclubfaceuvdt=norm(diff(CFunitvector));

== matlab function GolfSwing3D_KineticallyDrivenBlockCountStrip/LS Input Function/Left Shoulder Torque Output ==
  data: Time input; Killswitch input; LSInputXA parameter; LSInputYA parameter; LSInputZA parameter; LSInputXB parameter; LSInputYB parameter; LSInputZB parameter; LSPositionSetpointX parameter; LSPositionSetpointY parameter; GlobalGain parameter; JointTorqueLSX output; JointTorqueLSY output; JointTorqueLSZ output; LSDampeningX parameter; LSDampeningY parameter; LSDampeningZ parameter; LSConstantX parameter; LSConstantY parameter; LSConstantZ parameter; LSTimeGainX parameter; LSPositionGainY parameter; LSPositionGainZ parameter; LSPositionSetpointZ parameter; TargetLSPositionX parameter; TargetLSPositionY parameter; TargetLSPositionZ parameter; TargetLSVelocityX parameter; TargetLSVelocityY parameter; TargetLSVelocityZ parameter; LSPCGainX parameter; LSPCGainY parameter; LSPCGainZ parameter; LSVCGainX parameter; LSVCGainY parameter; LSVCGainZ parameter; ModelingMode parameter; ZVCFLSTorqueX parameter; ZVCFLSTorqueY parameter; ZVCFLSTorqueZ parameter; GlobalPCGain parameter; GlobalVCGain parameter; DampeningGlobalGain parameter; TargetImpactTime parameter; LSStartPositionX parameter; LSStartPositionY parameter; LSStartPositionZ parameter; LSStartVelocityX parameter; LSStartVelocityY parameter; LSStartVelocityZ parameter; LSPositionInputX output; LSPositionInputY output; LSPositionInputZ output; LSVelocityInputX output; LSVelocityInputY output; LSVelocityInputZ output; LSAccelerationInputX output; LSAccelerationInputY output; LSAccelerationInputZ output; LSAoX parameter; LSAoY parameter; LSAoZ parameter; KinematicMode parameter; LSInputYC parameter; LSInputXC parameter; LSInputZC parameter; LSTimeGainY parameter; LSTimeGainZ parameter; LSPositionX input; LSPositionY input; LSPositionZ input; LSVelocityX input; LSVelocityY input; LSVelocityZ input; LSPositionGainX parameter; LSAfX parameter; LSAfY parameter; LSAfZ parameter; LSInputXD parameter; LSInputXE parameter; LSInputXF parameter; LSInputXG parameter; LSInputYD parameter; LSInputYE parameter; LSInputYF parameter; LSInputYG parameter; LSInputZD parameter; LSInputZE parameter; LSInputZF parameter; LSInputZG parameter
function [JointTorqueLSX,JointTorqueLSY,JointTorqueLSZ,LSPositionInputX,LSPositionInputY,LSPositionInputZ,LSVelocityInputX,...
    LSVelocityInputY, LSVelocityInputZ,LSAccelerationInputX,LSAccelerationInputY,LSAccelerationInputZ] = fcn(Time,Killswitch, LSInputXA,LSInputYA,LSInputZA, LSInputXB,LSInputYB,LSInputZB, LSPositionSetpointX,LSPositionSetpointY,GlobalGain,...
    LSDampeningX, LSDampeningY, LSDampeningZ, LSConstantX, LSConstantY, LSConstantZ, LSTimeGainX, LSPositionGainY, LSPositionGainZ, LSPositionSetpointZ,...
    TargetLSPositionX, TargetLSPositionY, TargetLSPositionZ, TargetLSVelocityX, TargetLSVelocityY, TargetLSVelocityZ,LSPCGainX, LSPCGainY, LSPCGainZ, LSVCGainX,...
    LSVCGainY, LSVCGainZ,ModelingMode,ZVCFLSTorqueX, ZVCFLSTorqueY, ZVCFLSTorqueZ,GlobalPCGain, GlobalVCGain,DampeningGlobalGain,TargetImpactTime,LSStartPositionX,...
    LSStartPositionY, LSStartPositionZ, LSStartVelocityX, LSStartVelocityY, LSStartVelocityZ,LSAoX, LSAoY, LSAoZ, KinematicMode, LSInputYC, LSInputXC, LSInputZC,...
    LSTimeGainY, LSTimeGainZ, LSPositionX, LSPositionY, LSPositionZ, LSVelocityX, LSVelocityY,LSVelocityZ,...
    LSPositionGainX, LSAfX, LSAfY, LSAfZ,LSInputXD, LSInputXE, LSInputXF, LSInputXG,...
LSInputYD, LSInputYE, LSInputYF, LSInputYG, LSInputZD, LSInputZE, LSInputZF, LSInputZG)

%Tau=Time/TargetImpactTime;
t=Time;

% %%%%%%%%%%%%%%%%%%%%%%%%%%%%%%%%%%%%%%%%%%%
% % Kinetic Input Selection and Calculation
% %%%%%%%%%%%%%%%%%%%%%%%%%%%%%%%%%%%%%%%%%%%

if ModelingMode==0
    % Values are all set to zero.
    JointTorqueLSX=0;
    JointTorqueLSY=0;
    JointTorqueLSZ=0;
elseif ModelingMode==1
    % Control based strategy. Values are based on difference in value
    % between the current state and desired state.
    % LS Joint Rotational Deltas
    DeltaLSPositionX=LSPositionX-TargetLSPositionX;
    DeltaLSPositionY=LSPositionY-TargetLSPositionY;
    DeltaLSPositionZ=LSPositionZ-TargetLSPositionZ;
    DeltaLSVelocityX=LSVelocityX-TargetLSVelocityX;
    DeltaLSVelocityY=LSVelocityY-TargetLSVelocityY;
    DeltaLSVelocityZ=LSVelocityZ-TargetLSVelocityZ;
    % Control Based Strategy
    JointTorqueLSX=DeltaLSPositionX*LSPCGainX*GlobalPCGain-DeltaLSVelocityX*LSVCGainX*GlobalVCGain-DampeningGlobalGain*LSDampeningX*LSVelocityX;
    JointTorqueLSY=DeltaLSPositionY*LSPCGainY*GlobalPCGain-DeltaLSVelocityY*LSVCGainY*GlobalVCGain-DampeningGlobalGain*LSDampeningY*LSVelocityY;
    JointTorqueLSZ=DeltaLSPositionZ*LSPCGainZ*GlobalPCGain-DeltaLSVelocityZ*LSVCGainZ*GlobalVCGain-DampeningGlobalGain*LSDampeningZ*LSVelocityZ;
elseif ModelingMode==2
    % Forward Dynamics Based Strategy. Values are computed based on a
    % polynomial and a combination of dampening and position gained
    % factors.
    JointTorqueLSX=Killswitch*GlobalGain*(LSConstantX+LSTimeGainX*Time-LSPositionGainX*(LSPositionX-LSPositionSetpointX)...
    -LSDampeningX*LSVelocityX);
    JointTorqueLSY=Killswitch*GlobalGain*(LSConstantY+LSTimeGainY*Time-LSPositionGainY*(LSPositionY-LSPositionSetpointY)...
    -LSDampeningY*LSVelocityY);
    JointTorqueLSZ=Killswitch*GlobalGain*(LSConstantZ+LSTimeGainZ*Time-LSPositionGainZ*(LSPositionZ-LSPositionSetpointZ)...
    -LSDampeningZ*LSVelocityZ);
elseif ModelingMode==3
    JointTorqueLSX=HexPolyInputFunction(LSInputXA,LSInputXB,LSInputXC,LSInputXD,LSInputXE,LSInputXF,LSInputXG,Time)*Killswitch;
    JointTorqueLSY=HexPolyInputFunction(LSInputYA,LSInputYB,LSInputYC,LSInputYD,LSInputYE,LSInputYF,LSInputYG,Time)*Killswitch;
    JointTorqueLSZ=HexPolyInputFunction(LSInputZA,LSInputZB,LSInputZC,LSInputZD,LSInputZE,LSInputZF,LSInputZG,Time)*Killswitch;
else
    %ZVCF Based Joint Torques. Values are pulled from model workspace and
    %held constant.
    JointTorqueLSX=ZVCFLSTorqueX;
    JointTorqueLSY=ZVCFLSTorqueY;
    JointTorqueLSZ=ZVCFLSTorqueZ;
end

% %%%%%%%%%%%%%%%%%%%%%%%%%%%%%%%%%%%%%%%%%%%
% % Kinematic Input Selection and Calculation
% %%%%%%%%%%%%%%%%%%%%%%%%%%%%%%%%%%%%%%%%%%%

if KinematicMode==0
    % All kinematic values set to zero.
    LSPositionInputX=0;
    LSPositionInputY=0;
    LSPositionInputZ=0;
    LSVelocityInputX=0;
    LSVelocityInputY=0;
    LSVelocityInputZ=0;
    LSAccelerationInputX=0;
    LSAccelerationInputY=0;
    LSAccelerationInputZ=0;
elseif KinematicMode==1
    % 1st Order Acceleration, 2nd Order Velocity, 3rd Order Position Solution
    PTX=TargetLSPositionX;       
    VTX=TargetLSVelocityX;
    PTY=TargetLSPositionY;
    VTY=TargetLSVelocityY;
    PTZ=TargetLSPositionZ;
    VTZ=TargetLSVelocityZ;
    % Define Starting Position and Velocity
    PIX=LSStartPositionX;
    VIX=LSStartVelocityX;
    PIY=LSStartPositionY;
    VIY=LSStartVelocityY;
    PIZ=LSStartPositionZ;
    VIZ=LSStartVelocityZ;
    AX=3*((VTX+VIX)*TargetImpactTime-2*(PTX-PIX))/TargetImpactTime^3;         % Constant in position equation
    BX=-2*((VTX+2*VIX)*TargetImpactTime-3*(PTX-PIX))/TargetImpactTime^2;         % Constant in position equation
    CX=VIX;         % Starting Velocity at Time Zero
    DX=PIX;         % Starting Position at Time Zero
    AY=3*((VTY+VIY)*TargetImpactTime-2*(PTY-PIY))/TargetImpactTime^3;         % Constant in position equation
    BY=-2*((VTY+2*VIY)*TargetImpactTime-3*(PTY-PIY))/TargetImpactTime^2;         % Constant in position equation
    CY=VIY;         % Starting Velocity at Time Zero
    DY=PIY;         % Starting Position at Time Zero
    AZ=3*((VTZ+VIZ)*TargetImpactTime-2*(PTZ-PIZ))/TargetImpactTime^3;         % Constant in position equation
    BZ=-2*((VTZ+2*VIZ)*TargetImpactTime-3*(PTZ-PIZ))/TargetImpactTime^2;         % Constant in position equation
    CZ=VIZ;         % Starting Velocity at Time Zero
    DZ=PIZ;         % Starting Position at Time Zero
    % Equation for position as a function of time
    LSPositionInputX=AX*Time^3/3+BX*Time^2/2+CX*Time+DX;
    LSPositionInputY=AY*Time^3/3+BY*Time^2/2+CY*Time+DY;
    LSPositionInputZ=AZ*Time^3/3+BZ*Time^2/2+CZ*Time+DZ;
    LSVelocityInputX=AX*Time^2+BX*Time+CX;
    LSVelocityInputY=AY*Time^2+BY*Time+CY;
    LSVelocityInputZ=AZ*Time^2+BZ*Time+CZ;
    LSAccelerationInputX=2*AX*Time+BX;
    LSAccelerationInputY=2*AY*Time+BY;
    LSAccelerationInputZ=2*AZ*Time+BZ;
elseif KinematicMode==2
    % 2nd Order Acceleration, 3rd Order Velocity, 4th Order Position Solution
    Tt=TargetImpactTime;
    t=Time;
    PoX=LSStartPositionX;
    PoY=LSStartPositionY;
    PoZ=LSStartPositionZ;
    VoX=LSStartVelocityX;
    VoY=LSStartVelocityY;
    VoZ=LSStartVelocityZ;
    PfX=TargetLSPositionX;
    PfY=TargetLSPositionY;
    PfZ=TargetLSPositionZ;
    VfX=TargetLSVelocityX;
    VfY=TargetLSVelocityY;
    VfZ=TargetLSVelocityZ;
    AoX=LSAoX;
    AoY=LSAoY;
    AoZ=LSAoZ;
    LSPositionInputX=PoX + VoX*t + (AoX*t^2)/2 - (t^3*(4*PoX - 4*PfX + Tt*VfX + 3*Tt*VoX + AoX*Tt^2))/Tt^3 + (t^4*(6*PoX - 6*PfX + 2*Tt*VfX + 4*Tt*VoX + AoX*Tt^2))/(2*Tt^4);
    LSPositionInputY=PoY + VoY*t + (AoY*t^2)/2 - (t^3*(4*PoY - 4*PfY + Tt*VfY + 3*Tt*VoY + AoY*Tt^2))/Tt^3 + (t^4*(6*PoY - 6*PfY + 2*Tt*VfY + 4*Tt*VoY + AoY*Tt^2))/(2*Tt^4);
    LSPositionInputZ=PoZ + VoZ*t + (AoZ*t^2)/2 - (t^3*(4*PoZ - 4*PfZ + Tt*VfZ + 3*Tt*VoZ + AoZ*Tt^2))/Tt^3 + (t^4*(6*PoZ - 6*PfZ + 2*Tt*VfZ + 4*Tt*VoZ + AoZ*Tt^2))/(2*Tt^4);
    LSVelocityInputX=VoX + AoX*t - (3*t^2*(4*PoX - 4*PfX + Tt*VfX + 3*Tt*VoX + AoX*Tt^2))/Tt^3 + (2*t^3*(6*PoX - 6*PfX + 2*Tt*VfX + 4*Tt*VoX + AoX*Tt^2))/Tt^4;
    LSVelocityInputY=VoY + AoY*t - (3*t^2*(4*PoY - 4*PfY + Tt*VfY + 3*Tt*VoY + AoY*Tt^2))/Tt^3 + (2*t^3*(6*PoY - 6*PfY + 2*Tt*VfY + 4*Tt*VoY + AoY*Tt^2))/Tt^4;
    LSVelocityInputZ=VoZ + AoZ*t - (3*t^2*(4*PoZ - 4*PfZ + Tt*VfZ + 3*Tt*VoZ + AoZ*Tt^2))/Tt^3 + (2*t^3*(6*PoZ - 6*PfZ + 2*Tt*VfZ + 4*Tt*VoZ + AoZ*Tt^2))/Tt^4;
    LSAccelerationInputX=AoX + (6*t^2*(6*PoX - 6*PfX + 2*Tt*VfX + 4*Tt*VoX + AoX*Tt^2))/Tt^4 - (6*t*(4*PoX - 4*PfX + Tt*VfX + 3*Tt*VoX + AoX*Tt^2))/Tt^3;
    LSAccelerationInputY=AoY + (6*t^2*(6*PoY - 6*PfY + 2*Tt*VfY + 4*Tt*VoY + AoY*Tt^2))/Tt^4 - (6*t*(4*PoY - 4*PfY + Tt*VfY + 3*Tt*VoY + AoY*Tt^2))/Tt^3;
    LSAccelerationInputZ=AoZ + (6*t^2*(6*PoZ - 6*PfZ + 2*Tt*VfZ + 4*Tt*VoZ + AoZ*Tt^2))/Tt^4 - (6*t*(4*PoZ - 4*PfZ + Tt*VfZ + 3*Tt*VoZ + AoZ*Tt^2))/Tt^3;
else
    % 3rd Order Acceleration, 4th Order Velocity, 5th Order Position Solution
    Tt=TargetImpactTime;
    t=Time;
    PoX=LSStartPositionX;
    PoY=LSStartPositionY;
    PoZ=LSStartPositionZ;
    VoX=LSStartVelocityX;
    VoY=LSStartVelocityY;
    VoZ=LSStartVelocityZ;
    PfX=TargetLSPositionX;
    PfY=TargetLSPositionY;
    PfZ=TargetLSPositionZ;
    VfX=TargetLSVelocityX;
    VfY=TargetLSVelocityY;
    VfZ=TargetLSVelocityZ;
    AoX=LSAoX;
    AoY=LSAoY;
    AoZ=LSAoZ;
    AfX=LSAfX;
    AfY=LSAfY;
    AfZ=LSAfZ;
    LSPositionInputX=PoX+VoX*t+(AoX*t^2)/2-(t^5*(12*PoX-12*PfX+6*Tt*VfX+6*Tt*VoX-AfX*Tt^2+AoX*Tt^2))/(2*Tt^5)-(t^3*(20*PoX-20*PfX+8*Tt*VfX+12*Tt*VoX-AfX*Tt^2+3*AoX*Tt^2))/(2*Tt^3)+(t^4*(30*PoX-30*PfX+14*Tt*VfX+16*Tt*VoX-2*AfX*Tt^2+3*AoX*Tt^2))/(2*Tt^4);
    LSPositionInputY=PoY+VoY*t+(AoY*t^2)/2-(t^5*(12*PoY-12*PfY+6*Tt*VfY+6*Tt*VoY-AfY*Tt^2+AoY*Tt^2))/(2*Tt^5)-(t^3*(20*PoY-20*PfY+8*Tt*VfY+12*Tt*VoY-AfY*Tt^2+3*AoY*Tt^2))/(2*Tt^3)+(t^4*(30*PoY-30*PfY+14*Tt*VfY+16*Tt*VoY-2*AfY*Tt^2+3*AoY*Tt^2))/(2*Tt^4);  
    LSPositionInputZ=PoZ+VoZ*t+(AoZ*t^2)/2-(t^5*(12*PoZ-12*PfZ+6*Tt*VfZ+6*Tt*VoZ-AfZ*Tt^2+AoZ*Tt^2))/(2*Tt^5)-(t^3*(20*PoZ-20*PfZ+8*Tt*VfZ+12*Tt*VoZ-AfZ*Tt^2+3*AoZ*Tt^2))/(2*Tt^3)+(t^4*(30*PoZ-30*PfZ+14*Tt*VfZ+16*Tt*VoZ-2*AfZ*Tt^2+3*AoZ*Tt^2))/(2*Tt^4);
    LSVelocityInputX=VoX+AoX*t-(5*t^4*(12*PoX-12*PfX+6*Tt*VfX+6*Tt*VoX-AfX*Tt^2+AoX*Tt^2))/(2*Tt^5)-(3*t^2*(20*PoX-20*PfX+8*Tt*VfX+12*Tt*VoX-AfX*Tt^2+3*AoX*Tt^2))/(2*Tt^3)+(2*t^3*(30*PoX-30*PfX+14*Tt*VfX+16*Tt*VoX-2*AfX*Tt^2+3*AoX*Tt^2))/Tt^4;
    LSVelocityInputY=VoY+AoY*t-(5*t^4*(12*PoY-12*PfY+6*Tt*VfY+6*Tt*VoY-AfY*Tt^2+AoY*Tt^2))/(2*Tt^5)-(3*t^2*(20*PoY-20*PfY+8*Tt*VfY+12*Tt*VoY-AfY*Tt^2+3*AoY*Tt^2))/(2*Tt^3)+(2*t^3*(30*PoY-30*PfY+14*Tt*VfY+16*Tt*VoY-2*AfY*Tt^2+3*AoY*Tt^2))/Tt^4;
    LSVelocityInputZ=VoZ+AoZ*t-(5*t^4*(12*PoZ-12*PfZ+6*Tt*VfZ+6*Tt*VoZ-AfZ*Tt^2+AoZ*Tt^2))/(2*Tt^5)-(3*t^2*(20*PoZ-20*PfZ+8*Tt*VfZ+12*Tt*VoZ-AfZ*Tt^2+3*AoZ*Tt^2))/(2*Tt^3)+(2*t^3*(30*PoZ-30*PfZ+14*Tt*VfZ+16*Tt*VoZ-2*AfZ*Tt^2+3*AoZ*Tt^2))/Tt^4;
    LSAccelerationInputX=AoX-(3*t*(20*PoX-20*PfX+8*Tt*VfX+12*Tt*VoX-AfX*Tt^2+3*AoX*Tt^2))/Tt^3-(10*t^3*(12*PoX-12*PfX+6*Tt*VfX+6*Tt*VoX-AfX*Tt^2+AoX*Tt^2))/Tt^5+(6*t^2*(30*PoX-30*PfX+14*Tt*VfX+16*Tt*VoX-2*AfX*Tt^2+3*AoX*Tt^2))/Tt^4;
    LSAccelerationInputY=AoY-(3*t*(20*PoY-20*PfY+8*Tt*VfY+12*Tt*VoY-AfY*Tt^2+3*AoY*Tt^2))/Tt^3-(10*t^3*(12*PoY-12*PfY+6*Tt*VfY+6*Tt*VoY-AfY*Tt^2+AoY*Tt^2))/Tt^5+(6*t^2*(30*PoY-30*PfY+14*Tt*VfY+16*Tt*VoY-2*AfY*Tt^2+3*AoY*Tt^2))/Tt^4;
    LSAccelerationInputZ=AoZ-(3*t*(20*PoZ-20*PfZ+8*Tt*VfZ+12*Tt*VoZ-AfZ*Tt^2+3*AoZ*Tt^2))/Tt^3-(10*t^3*(12*PoZ-12*PfZ+6*Tt*VfZ+6*Tt*VoZ-AfZ*Tt^2+AoZ*Tt^2))/Tt^5+(6*t^2*(30*PoZ-30*PfZ+14*Tt*VfZ+16*Tt*VoZ-2*AfZ*Tt^2+3*AoZ*Tt^2))/Tt^4;
end


% Calculate Higher Order Derivatives of the Position Outputs
LSJerkX=gradient(LSAccelerationInputX,t);
LSJerkY=gradient(LSAccelerationInputY,t);
LSJerkZ=gradient(LSAccelerationInputZ,t);
LSSnapX=gradient(LSJerkX,t);
LSSnapY=gradient(LSJerkY,t);
LSSnapZ=gradient(LSJerkZ,t);
LSCrackleX=gradient(LSSnapX,t);
LSCrackleY=gradient(LSSnapY,t);
LSCrackleZ=gradient(LSSnapZ,t);
LSPopX=gradient(LSCrackleX,t);
LSPopY=gradient(LSCrackleY,t);
LSPopZ=gradient(LSCrackleZ,t);
